simulink model "xz_low_speed_control"  (R2020a)
settings: Solver=VariableStepAuto  StartTime=0.0  StopTime=10.0  RelTol=1e-3
settings Model: Creator=Tamer  LastModifiedBy=Tamer

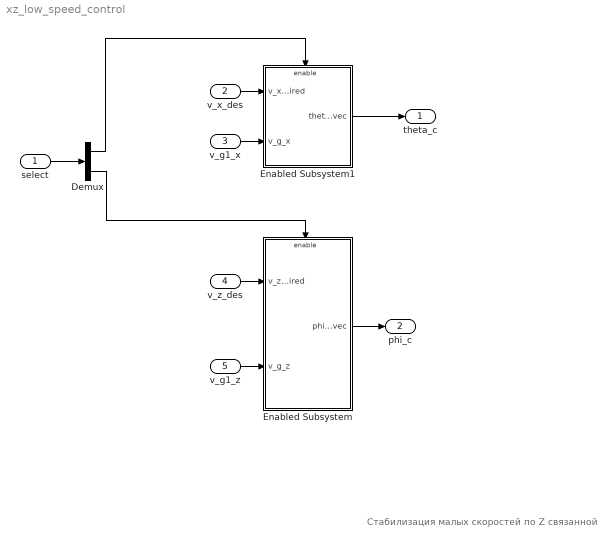
== system xz_low_speed_control ==
  note: Стабилизация малых скоростей по Z связанной
  select : Inport
  v_x_des : Inport  Port=2
  v_g1_x : Inport  Port=3
  v_z_des : Inport  Port=4
  v_g1_z : Inport  Port=5
  Demux : Demux  Outputs=2
  Enabled Subsystem : Subsystem  TreatAsAtomicUnit=on
  Enabled Subsystem1 : Subsystem  TreatAsAtomicUnit=on
  theta_c : Outport
  phi_c : Outport  Port=2
  wires:
  Enabled Subsystem/1(phi_c_vec) -> phi_c/1
  select/1 -> Demux/1
  Demux/2 -> Enabled Subsystem/Enable
  Enabled Subsystem1/1(theta_c_vec) -> theta_c/1
  Demux/1 -> Enabled Subsystem1/Enable
  v_g1_z/1 -> Enabled Subsystem/2(v_g_z)
  v_z_des/1 -> Enabled Subsystem/1(v_z_desired)
  v_g1_x/1 -> Enabled Subsystem1/2(v_g_x)
  v_x_des/1 -> Enabled Subsystem1/1(v_x_desired)

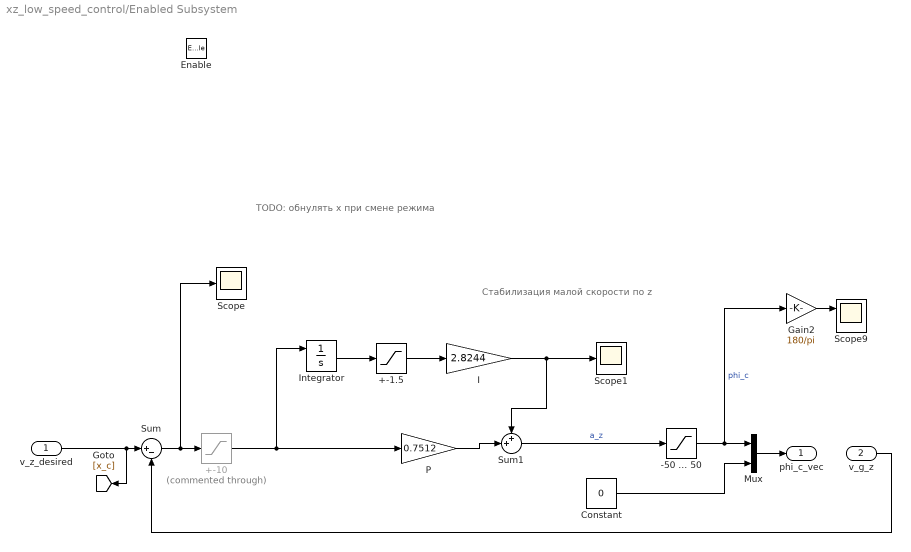
== system xz_low_speed_control/Enabled Subsystem ==
  note: TODO: обнулять x при смене режима
  note: Стабилизация малой скорости по z
  v_z_desired : Inport
  v_g_z : Inport  Port=2
  Enable : EnablePort
  "+-1.5 " : Saturate
  +-10 : Saturate  Commented=through  UpperLimit=10  LowerLimit=-10
  -50 ... 50 : Saturate  UpperLimit=deg2rad(50)  LowerLimit=deg2rad(-50)
  Constant : Constant  Value=0
  Gain2 : Gain  Gain=180/pi
  I : Gain  Gain=2.8244
  Integrator : Integrator  ExternalReset=either
  Mux : Mux  Inputs=2
  P : Gain  Gain=0.7512
  Scope : Scope
  Scope1 : Scope
  Scope9 : Scope  NumInputPorts=2
  Sum : Sum  Inputs=|+-
  Sum1 : Sum  Inputs=++|
  phi_c_vec : Outport
  wires:
  v_g_z/1 -> Sum/2
  Integrator/1 -> "+-1.5 "/1
  "+-1.5 "/1 -> I/1
  I/1 -> Sum1/1, Scope1/1
  Sum1/1 -> -50 ... 50/1  "a_z"
  Sum/1 -> Scope/1, +-10/1
  Constant/1 -> Mux/2
  v_z_desired/1 -> [x_c], Sum/1
  -50 ... 50/1 -> Gain2/1, Mux/1  "phi_c"
  +-10/1 -> P/1, Integrator/1
  Mux/1 -> phi_c_vec/1
  P/1 -> Sum1/2
  Gain2/1 -> Scope9/1

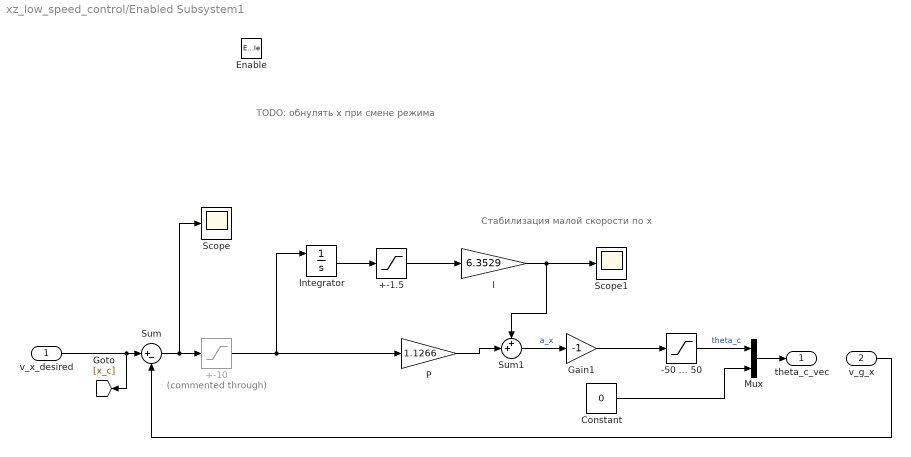
== system xz_low_speed_control/Enabled Subsystem1 ==
  note: TODO: обнулять x при смене режима
  note: Стабилизация малой скорости по х
  v_x_desired : Inport
  v_g_x : Inport  Port=2
  Enable : EnablePort
  "+-1.5 " : Saturate
  +-10 : Saturate  Commented=through  UpperLimit=10  LowerLimit=-10
  -50 ... 50 : Saturate  UpperLimit=deg2rad(50)  LowerLimit=deg2rad(-50)
  Constant : Constant  Value=0
  Gain1 : Gain  Gain=-1
  I : Gain  Gain=6.3529
  Integrator : Integrator  ExternalReset=either
  Mux : Mux  Inputs=2
  P : Gain  Gain=1.1266
  Scope : Scope
  Scope1 : Scope
  Sum : Sum  Inputs=|+-
  Sum1 : Sum  Inputs=++|
  theta_c_vec : Outport
  wires:
  Sum/1 -> Scope/1, +-10/1
  -50 ... 50/1 -> Mux/1  "theta_c"
  Sum1/1 -> Gain1/1  "a_x"
  "+-1.5 "/1 -> I/1
  Integrator/1 -> "+-1.5 "/1
  v_x_desired/1 -> [x_c], Sum/1
  v_g_x/1 -> Sum/2
  Constant/1 -> Mux/2
  +-10/1 -> P/1, Integrator/1
  Mux/1 -> theta_c_vec/1
  Gain1/1 -> -50 ... 50/1
  P/1 -> Sum1/2
  I/1 -> Sum1/1, Scope1/1
